simulink model "AutonomousModel_V3"  (R2020b)
settings: Solver=ode23t  StartTime=0.0  StopTime=180.1  FixedStep=0.05  RelTol=1e-3  EnableMultiTasking=on
model workspace (MAT data in the model file):
  mapForSim : object (value not decoded)
  occGrid : robotics.BinaryOccupancyGrid (value not decoded)
undefined symbols (not defined in the file): cellLevel, cellPose, cellTypeArray, FloorSurface, isoPoses, platformPoses, PlowSurface, Ref, RobotSurface, WallSurface, X, Y, Z
libraries: sm_lib x286, nesl_utility x157, simulink x72, pid_lib x3
(part 14 of 14)

== matlab function AutonomousModel_V3/BEST Robotics 2020 Game (Double-Click)/Cells/Object9/MATLAB Function ==
  settings: updateMethod=DISCRETE
  data: latch input; scoreLevel input; inuse input; target input; time input; objPoseX output; robotPoseX input; robotPoseY input; objPoseY output; latched output; initPose parameter; objId parameter; cellType output; endType output; cellTypeArray parameter; gameTime parameter; platformPoses parameter; cellLevel parameter
function [objPoseX, objPoseY, latched, cellType,endType] = latchObject(latch,scoreLevel, inuse, target, time, robotPoseX, robotPoseY, initPose, objId, cellTypeArray, gameTime, platformPoses, cellLevel)
persistent stateX stateY level pickup
if isempty(stateX)
    stateX=initPose(1);
    stateY=initPose(2);
    level=cellLevel;
    pickup=0;
end

if ~latch
     pickup=0;
    if level && ((stateX > platformPoses(1,1)-0.21 && stateX < platformPoses(1,1)+0.21...
            && stateY > platformPoses(1,2)-0.21 && stateY < platformPoses(1,2) +0.21) || ...
            (stateX > platformPoses(2,1)-0.21 && stateX < platformPoses(2,1)+0.21...
            && stateY > platformPoses(2,2)-0.21 && stateY < platformPoses(2,2) +0.21))
        latched=0.4;
    else
        level=0;
        latched=0;
    end
elseif pickup
    stateX=robotPoseX;
    stateY=robotPoseY;
    level=scoreLevel;
    latched=0.15 +level*0.4;
elseif ~inuse && latch && target == objId && ...
        sqrt((stateX-robotPoseX)^2+(stateY-robotPoseY)^2) < 0.08 && scoreLevel==level
    
        pickup=1;
        latched=0.15;
else
   if level && ((stateX > platformPoses(1,1)-0.21 && stateX < platformPoses(1,1)+0.21...
            && stateY > platformPoses(1,2)-0.21 && stateY < platformPoses(1,2) +0.21) || ...
            (stateX > platformPoses(2,1)-0.21 && stateX < platformPoses(2,1)+0.21...
            && stateY > platformPoses(2,2)-0.21 && stateY < platformPoses(2,2) +0.21))
        latched=0.4;
    else
        level=0;
        latched=0;
    end
end
if sqrt((stateX-robotPoseX)^2+(stateY-robotPoseY)^2) < 0.1 && scoreLevel==level
    cellType=cellTypeArray(objId);
else
    cellType=nan;
end

if time > gameTime
    endType=cellTypeArray(objId)+1;
else
    endType=0;
end

objPoseX=stateX;
objPoseY=stateY;

== stateflow chart AutonomousModel_V3/Stateflow ==
  state DROP_1
    entry: dropVac = [1 0 0]
  state DROP_2
    entry: dropVac = [0 1 1]
  state DROP_3
    entry: dropVac = [0 0 1]
  (default) -> DROP_1
  DROP_1 -> DROP_2 : after(1, sec)
  DROP_2 -> DROP_3 : after(1, sec)
  data: dropVac output

== stateflow chart AutonomousModel_V3/Simulink Function2/Stateflow2 ==
  state SETTLE
  state RESET_MOTORS
    entry:
    leftMotor = 0
    rightMotor = 0
  (default) -> SETTLE
  RESET_MOTORS -> SETTLE
  SETTLE -> RESET_MOTORS : [angleHasSettled]
  data: angleHasSettled input; leftMotor data_store_memory; rightMotor data_store_memory

== matlab function AutonomousModel_V3/BEST Robotics 2020 Game (Double-Click)/Cells/Object10/MATLAB Function ==
  settings: updateMethod=DISCRETE
  data: latch input; scoreLevel input; inuse input; target input; time input; objPoseX output; robotPoseX input; robotPoseY input; objPoseY output; latched output; initPose parameter; objId parameter; cellType output; endType output; cellTypeArray parameter; gameTime parameter; platformPoses parameter; cellLevel parameter
function [objPoseX, objPoseY, latched, cellType,endType] = latchObject(latch,scoreLevel, inuse, target, time, robotPoseX, robotPoseY, initPose, objId, cellTypeArray, gameTime, platformPoses, cellLevel)
persistent stateX stateY level pickup
if isempty(stateX)
    stateX=initPose(1);
    stateY=initPose(2);
    level=cellLevel;
    pickup=0;
end

if ~latch
     pickup=0;
    if level && ((stateX > platformPoses(1,1)-0.21 && stateX < platformPoses(1,1)+0.21...
            && stateY > platformPoses(1,2)-0.21 && stateY < platformPoses(1,2) +0.21) || ...
            (stateX > platformPoses(2,1)-0.21 && stateX < platformPoses(2,1)+0.21...
            && stateY > platformPoses(2,2)-0.21 && stateY < platformPoses(2,2) +0.21))
        latched=0.4;
    else
        level=0;
        latched=0;
    end
elseif pickup
    stateX=robotPoseX;
    stateY=robotPoseY;
    level=scoreLevel;
    latched=0.15 +level*0.4;
elseif ~inuse && latch && target == objId && ...
        sqrt((stateX-robotPoseX)^2+(stateY-robotPoseY)^2) < 0.08 && scoreLevel==level
    
        pickup=1;
        latched=0.15;
else
   if level && ((stateX > platformPoses(1,1)-0.21 && stateX < platformPoses(1,1)+0.21...
            && stateY > platformPoses(1,2)-0.21 && stateY < platformPoses(1,2) +0.21) || ...
            (stateX > platformPoses(2,1)-0.21 && stateX < platformPoses(2,1)+0.21...
            && stateY > platformPoses(2,2)-0.21 && stateY < platformPoses(2,2) +0.21))
        latched=0.4;
    else
        level=0;
        latched=0;
    end
end
if sqrt((stateX-robotPoseX)^2+(stateY-robotPoseY)^2) < 0.1 && scoreLevel==level
    cellType=cellTypeArray(objId);
else
    cellType=nan;
end

if time > gameTime
    endType=cellTypeArray(objId)+1;
else
    endType=0;
end

objPoseX=stateX;
objPoseY=stateY;

== matlab function AutonomousModel_V3/BEST Robotics 2020 Game (Double-Click)/Cells/Object11/MATLAB Function ==
  settings: updateMethod=DISCRETE
  data: latch input; scoreLevel input; inuse input; target input; time input; objPoseX output; robotPoseX input; robotPoseY input; objPoseY output; latched output; initPose parameter; objId parameter; cellType output; endType output; cellTypeArray parameter; gameTime parameter; platformPoses parameter; cellLevel parameter
function [objPoseX, objPoseY, latched, cellType,endType] = latchObject(latch,scoreLevel, inuse, target, time, robotPoseX, robotPoseY, initPose, objId, cellTypeArray, gameTime, platformPoses, cellLevel)
persistent stateX stateY level pickup
if isempty(stateX)
    stateX=initPose(1);
    stateY=initPose(2);
    level=cellLevel;
    pickup=0;
end

if ~latch
     pickup=0;
    if level && ((stateX > platformPoses(1,1)-0.21 && stateX < platformPoses(1,1)+0.21...
            && stateY > platformPoses(1,2)-0.21 && stateY < platformPoses(1,2) +0.21) || ...
            (stateX > platformPoses(2,1)-0.21 && stateX < platformPoses(2,1)+0.21...
            && stateY > platformPoses(2,2)-0.21 && stateY < platformPoses(2,2) +0.21))
        latched=0.4;
    else
        level=0;
        latched=0;
    end
elseif pickup
    stateX=robotPoseX;
    stateY=robotPoseY;
    level=scoreLevel;
    latched=0.15 +level*0.4;
elseif ~inuse && latch && target == objId && ...
        sqrt((stateX-robotPoseX)^2+(stateY-robotPoseY)^2) < 0.08 && scoreLevel==level
    
        pickup=1;
        latched=0.15;
else
   if level && ((stateX > platformPoses(1,1)-0.21 && stateX < platformPoses(1,1)+0.21...
            && stateY > platformPoses(1,2)-0.21 && stateY < platformPoses(1,2) +0.21) || ...
            (stateX > platformPoses(2,1)-0.21 && stateX < platformPoses(2,1)+0.21...
            && stateY > platformPoses(2,2)-0.21 && stateY < platformPoses(2,2) +0.21))
        latched=0.4;
    else
        level=0;
        latched=0;
    end
end
if sqrt((stateX-robotPoseX)^2+(stateY-robotPoseY)^2) < 0.1 && scoreLevel==level
    cellType=cellTypeArray(objId);
else
    cellType=nan;
end

if time > gameTime
    endType=cellTypeArray(objId)+1;
else
    endType=0;
end

objPoseX=stateX;
objPoseY=stateY;

== matlab function AutonomousModel_V3/BEST Robotics 2020 Game (Double-Click)/Cells/Object12/MATLAB Function ==
  settings: updateMethod=DISCRETE
  data: latch input; scoreLevel input; inuse input; target input; time input; objPoseX output; robotPoseX input; robotPoseY input; objPoseY output; latched output; initPose parameter; objId parameter; cellType output; endType output; cellTypeArray parameter; gameTime parameter; platformPoses parameter; cellLevel parameter
function [objPoseX, objPoseY, latched, cellType,endType] = latchObject(latch,scoreLevel, inuse, target, time, robotPoseX, robotPoseY, initPose, objId, cellTypeArray, gameTime, platformPoses, cellLevel)
persistent stateX stateY level pickup
if isempty(stateX)
    stateX=initPose(1);
    stateY=initPose(2);
    level=cellLevel;
    pickup=0;
end

if ~latch
     pickup=0;
    if level && ((stateX > platformPoses(1,1)-0.21 && stateX < platformPoses(1,1)+0.21...
            && stateY > platformPoses(1,2)-0.21 && stateY < platformPoses(1,2) +0.21) || ...
            (stateX > platformPoses(2,1)-0.21 && stateX < platformPoses(2,1)+0.21...
            && stateY > platformPoses(2,2)-0.21 && stateY < platformPoses(2,2) +0.21))
        latched=0.4;
    else
        level=0;
        latched=0;
    end
elseif pickup
    stateX=robotPoseX;
    stateY=robotPoseY;
    level=scoreLevel;
    latched=0.15 +level*0.4;
elseif ~inuse && latch && target == objId && ...
        sqrt((stateX-robotPoseX)^2+(stateY-robotPoseY)^2) < 0.08 && scoreLevel==level
    
        pickup=1;
        latched=0.15;
else
   if level && ((stateX > platformPoses(1,1)-0.21 && stateX < platformPoses(1,1)+0.21...
            && stateY > platformPoses(1,2)-0.21 && stateY < platformPoses(1,2) +0.21) || ...
            (stateX > platformPoses(2,1)-0.21 && stateX < platformPoses(2,1)+0.21...
            && stateY > platformPoses(2,2)-0.21 && stateY < platformPoses(2,2) +0.21))
        latched=0.4;
    else
        level=0;
        latched=0;
    end
end
if sqrt((stateX-robotPoseX)^2+(stateY-robotPoseY)^2) < 0.1 && scoreLevel==level
    cellType=cellTypeArray(objId);
else
    cellType=nan;
end

if time > gameTime
    endType=cellTypeArray(objId)+1;
else
    endType=0;
end

objPoseX=stateX;
objPoseY=stateY;

== matlab function AutonomousModel_V3/BEST Robotics 2020 Game (Double-Click)/Cells/Object13/MATLAB Function ==
  settings: updateMethod=DISCRETE
  data: latch input; scoreLevel input; inuse input; target input; time input; objPoseX output; robotPoseX input; robotPoseY input; objPoseY output; latched output; initPose parameter; objId parameter; cellType output; endType output; cellTypeArray parameter; gameTime parameter; platformPoses parameter; cellLevel parameter
function [objPoseX, objPoseY, latched, cellType,endType] = latchObject(latch,scoreLevel, inuse, target, time, robotPoseX, robotPoseY, initPose, objId, cellTypeArray, gameTime, platformPoses, cellLevel)
persistent stateX stateY level pickup
if isempty(stateX)
    stateX=initPose(1);
    stateY=initPose(2);
    level=cellLevel;
    pickup=0;
end

if ~latch
     pickup=0;
    if level && ((stateX > platformPoses(1,1)-0.21 && stateX < platformPoses(1,1)+0.21...
            && stateY > platformPoses(1,2)-0.21 && stateY < platformPoses(1,2) +0.21) || ...
            (stateX > platformPoses(2,1)-0.21 && stateX < platformPoses(2,1)+0.21...
            && stateY > platformPoses(2,2)-0.21 && stateY < platformPoses(2,2) +0.21))
        latched=0.4;
    else
        level=0;
        latched=0;
    end
elseif pickup
    stateX=robotPoseX;
    stateY=robotPoseY;
    level=scoreLevel;
    latched=0.15 +level*0.4;
elseif ~inuse && latch && target == objId && ...
        sqrt((stateX-robotPoseX)^2+(stateY-robotPoseY)^2) < 0.08 && scoreLevel==level
    
        pickup=1;
        latched=0.15;
else
   if level && ((stateX > platformPoses(1,1)-0.21 && stateX < platformPoses(1,1)+0.21...
            && stateY > platformPoses(1,2)-0.21 && stateY < platformPoses(1,2) +0.21) || ...
            (stateX > platformPoses(2,1)-0.21 && stateX < platformPoses(2,1)+0.21...
            && stateY > platformPoses(2,2)-0.21 && stateY < platformPoses(2,2) +0.21))
        latched=0.4;
    else
        level=0;
        latched=0;
    end
end
if sqrt((stateX-robotPoseX)^2+(stateY-robotPoseY)^2) < 0.1 && scoreLevel==level
    cellType=cellTypeArray(objId);
else
    cellType=nan;
end

if time > gameTime
    endType=cellTypeArray(objId)+1;
else
    endType=0;
end

objPoseX=stateX;
objPoseY=stateY;

== matlab function AutonomousModel_V3/BEST Robotics 2020 Game (Double-Click)/Cells/Object14/MATLAB Function ==
  settings: updateMethod=DISCRETE
  data: latch input; scoreLevel input; inuse input; target input; time input; objPoseX output; robotPoseX input; robotPoseY input; objPoseY output; latched output; initPose parameter; objId parameter; cellType output; endType output; cellTypeArray parameter; gameTime parameter; platformPoses parameter; cellLevel parameter
function [objPoseX, objPoseY, latched, cellType,endType] = latchObject(latch,scoreLevel, inuse, target, time, robotPoseX, robotPoseY, initPose, objId, cellTypeArray, gameTime, platformPoses, cellLevel)
persistent stateX stateY level pickup
if isempty(stateX)
    stateX=initPose(1);
    stateY=initPose(2);
    level=cellLevel;
    pickup=0;
end

if ~latch
     pickup=0;
    if level && ((stateX > platformPoses(1,1)-0.21 && stateX < platformPoses(1,1)+0.21...
            && stateY > platformPoses(1,2)-0.21 && stateY < platformPoses(1,2) +0.21) || ...
            (stateX > platformPoses(2,1)-0.21 && stateX < platformPoses(2,1)+0.21...
            && stateY > platformPoses(2,2)-0.21 && stateY < platformPoses(2,2) +0.21))
        latched=0.4;
    else
        level=0;
        latched=0;
    end
elseif pickup
    stateX=robotPoseX;
    stateY=robotPoseY;
    level=scoreLevel;
    latched=0.15 +level*0.4;
elseif ~inuse && latch && target == objId && ...
        sqrt((stateX-robotPoseX)^2+(stateY-robotPoseY)^2) < 0.08 && scoreLevel==level
    
        pickup=1;
        latched=0.15;
else
   if level && ((stateX > platformPoses(1,1)-0.21 && stateX < platformPoses(1,1)+0.21...
            && stateY > platformPoses(1,2)-0.21 && stateY < platformPoses(1,2) +0.21) || ...
            (stateX > platformPoses(2,1)-0.21 && stateX < platformPoses(2,1)+0.21...
            && stateY > platformPoses(2,2)-0.21 && stateY < platformPoses(2,2) +0.21))
        latched=0.4;
    else
        level=0;
        latched=0;
    end
end
if sqrt((stateX-robotPoseX)^2+(stateY-robotPoseY)^2) < 0.1 && scoreLevel==level
    cellType=cellTypeArray(objId);
else
    cellType=nan;
end

if time > gameTime
    endType=cellTypeArray(objId)+1;
else
    endType=0;
end

objPoseX=stateX;
objPoseY=stateY;

== matlab function AutonomousModel_V3/BEST Robotics 2020 Game (Double-Click)/Cells/Object15/MATLAB Function ==
  settings: updateMethod=DISCRETE
  data: latch input; scoreLevel input; inuse input; target input; time input; objPoseX output; robotPoseX input; robotPoseY input; objPoseY output; latched output; initPose parameter; objId parameter; cellType output; endType output; cellTypeArray parameter; gameTime parameter; platformPoses parameter; cellLevel parameter
function [objPoseX, objPoseY, latched, cellType,endType] = latchObject(latch,scoreLevel, inuse, target, time, robotPoseX, robotPoseY, initPose, objId, cellTypeArray, gameTime, platformPoses, cellLevel)
persistent stateX stateY level pickup
if isempty(stateX)
    stateX=initPose(1);
    stateY=initPose(2);
    level=cellLevel;
    pickup=0;
end

if ~latch
     pickup=0;
    if level && ((stateX > platformPoses(1,1)-0.21 && stateX < platformPoses(1,1)+0.21...
            && stateY > platformPoses(1,2)-0.21 && stateY < platformPoses(1,2) +0.21) || ...
            (stateX > platformPoses(2,1)-0.21 && stateX < platformPoses(2,1)+0.21...
            && stateY > platformPoses(2,2)-0.21 && stateY < platformPoses(2,2) +0.21))
        latched=0.4;
    else
        level=0;
        latched=0;
    end
elseif pickup
    stateX=robotPoseX;
    stateY=robotPoseY;
    level=scoreLevel;
    latched=0.15 +level*0.4;
elseif ~inuse && latch && target == objId && ...
        sqrt((stateX-robotPoseX)^2+(stateY-robotPoseY)^2) < 0.08 && scoreLevel==level
    
        pickup=1;
        latched=0.15;
else
   if level && ((stateX > platformPoses(1,1)-0.21 && stateX < platformPoses(1,1)+0.21...
            && stateY > platformPoses(1,2)-0.21 && stateY < platformPoses(1,2) +0.21) || ...
            (stateX > platformPoses(2,1)-0.21 && stateX < platformPoses(2,1)+0.21...
            && stateY > platformPoses(2,2)-0.21 && stateY < platformPoses(2,2) +0.21))
        latched=0.4;
    else
        level=0;
        latched=0;
    end
end
if sqrt((stateX-robotPoseX)^2+(stateY-robotPoseY)^2) < 0.1 && scoreLevel==level
    cellType=cellTypeArray(objId);
else
    cellType=nan;
end

if time > gameTime
    endType=cellTypeArray(objId)+1;
else
    endType=0;
end

objPoseX=stateX;
objPoseY=stateY;

== matlab function AutonomousModel_V3/BEST Robotics 2020 Game (Double-Click)/Cells/Object16/MATLAB Function ==
  settings: updateMethod=DISCRETE
  data: latch input; scoreLevel input; inuse input; target input; time input; objPoseX output; robotPoseX input; robotPoseY input; objPoseY output; latched output; initPose parameter; objId parameter; cellType output; endType output; cellTypeArray parameter; gameTime parameter; platformPoses parameter; cellLevel parameter
function [objPoseX, objPoseY, latched, cellType,endType] = latchObject(latch,scoreLevel, inuse, target, time, robotPoseX, robotPoseY, initPose, objId, cellTypeArray, gameTime, platformPoses, cellLevel)
persistent stateX stateY level pickup
if isempty(stateX)
    stateX=initPose(1);
    stateY=initPose(2);
    level=cellLevel;
    pickup=0;
end

if ~latch
     pickup=0;
    if level && ((stateX > platformPoses(1,1)-0.21 && stateX < platformPoses(1,1)+0.21...
            && stateY > platformPoses(1,2)-0.21 && stateY < platformPoses(1,2) +0.21) || ...
            (stateX > platformPoses(2,1)-0.21 && stateX < platformPoses(2,1)+0.21...
            && stateY > platformPoses(2,2)-0.21 && stateY < platformPoses(2,2) +0.21))
        latched=0.4;
    else
        level=0;
        latched=0;
    end
elseif pickup
    stateX=robotPoseX;
    stateY=robotPoseY;
    level=scoreLevel;
    latched=0.15 +level*0.4;
elseif ~inuse && latch && target == objId && ...
        sqrt((stateX-robotPoseX)^2+(stateY-robotPoseY)^2) < 0.08 && scoreLevel==level
    
        pickup=1;
        latched=0.15;
else
   if level && ((stateX > platformPoses(1,1)-0.21 && stateX < platformPoses(1,1)+0.21...
            && stateY > platformPoses(1,2)-0.21 && stateY < platformPoses(1,2) +0.21) || ...
            (stateX > platformPoses(2,1)-0.21 && stateX < platformPoses(2,1)+0.21...
            && stateY > platformPoses(2,2)-0.21 && stateY < platformPoses(2,2) +0.21))
        latched=0.4;
    else
        level=0;
        latched=0;
    end
end
if sqrt((stateX-robotPoseX)^2+(stateY-robotPoseY)^2) < 0.1 && scoreLevel==level
    cellType=cellTypeArray(objId);
else
    cellType=nan;
end

if time > gameTime
    endType=cellTypeArray(objId)+1;
else
    endType=0;
end

objPoseX=stateX;
objPoseY=stateY;

== matlab function AutonomousModel_V3/BEST Robotics 2020 Game (Double-Click)/Cells/Object17/MATLAB Function ==
  settings: updateMethod=DISCRETE
  data: latch input; scoreLevel input; inuse input; target input; time input; objPoseX output; robotPoseX input; robotPoseY input; objPoseY output; latched output; initPose parameter; objId parameter; cellType output; endType output; cellTypeArray parameter; gameTime parameter; platformPoses parameter; cellLevel parameter
function [objPoseX, objPoseY, latched, cellType,endType] = latchObject(latch,scoreLevel, inuse, target, time, robotPoseX, robotPoseY, initPose, objId, cellTypeArray, gameTime, platformPoses, cellLevel)
persistent stateX stateY level pickup
if isempty(stateX)
    stateX=initPose(1);
    stateY=initPose(2);
    level=cellLevel;
    pickup=0;
end

if ~latch
     pickup=0;
    if level && ((stateX > platformPoses(1,1)-0.21 && stateX < platformPoses(1,1)+0.21...
            && stateY > platformPoses(1,2)-0.21 && stateY < platformPoses(1,2) +0.21) || ...
            (stateX > platformPoses(2,1)-0.21 && stateX < platformPoses(2,1)+0.21...
            && stateY > platformPoses(2,2)-0.21 && stateY < platformPoses(2,2) +0.21))
        latched=0.4;
    else
        level=0;
        latched=0;
    end
elseif pickup
    stateX=robotPoseX;
    stateY=robotPoseY;
    level=scoreLevel;
    latched=0.15 +level*0.4;
elseif ~inuse && latch && target == objId && ...
        sqrt((stateX-robotPoseX)^2+(stateY-robotPoseY)^2) < 0.08 && scoreLevel==level
    
        pickup=1;
        latched=0.15;
else
   if level && ((stateX > platformPoses(1,1)-0.21 && stateX < platformPoses(1,1)+0.21...
            && stateY > platformPoses(1,2)-0.21 && stateY < platformPoses(1,2) +0.21) || ...
            (stateX > platformPoses(2,1)-0.21 && stateX < platformPoses(2,1)+0.21...
            && stateY > platformPoses(2,2)-0.21 && stateY < platformPoses(2,2) +0.21))
        latched=0.4;
    else
        level=0;
        latched=0;
    end
end
if sqrt((stateX-robotPoseX)^2+(stateY-robotPoseY)^2) < 0.1 && scoreLevel==level
    cellType=cellTypeArray(objId);
else
    cellType=nan;
end

if time > gameTime
    endType=cellTypeArray(objId)+1;
else
    endType=0;
end

objPoseX=stateX;
objPoseY=stateY;

== matlab function AutonomousModel_V3/BEST Robotics 2020 Game (Double-Click)/Cells/Object18/MATLAB Function ==
  settings: updateMethod=DISCRETE
  data: latch input; scoreLevel input; inuse input; target input; time input; objPoseX output; robotPoseX input; robotPoseY input; objPoseY output; latched output; initPose parameter; objId parameter; cellType output; endType output; cellTypeArray parameter; gameTime parameter; platformPoses parameter; cellLevel parameter
function [objPoseX, objPoseY, latched, cellType,endType] = latchObject(latch,scoreLevel, inuse, target, time, robotPoseX, robotPoseY, initPose, objId, cellTypeArray, gameTime, platformPoses, cellLevel)
persistent stateX stateY level pickup
if isempty(stateX)
    stateX=initPose(1);
    stateY=initPose(2);
    level=cellLevel;
    pickup=0;
end

if ~latch
     pickup=0;
    if level && ((stateX > platformPoses(1,1)-0.21 && stateX < platformPoses(1,1)+0.21...
            && stateY > platformPoses(1,2)-0.21 && stateY < platformPoses(1,2) +0.21) || ...
            (stateX > platformPoses(2,1)-0.21 && stateX < platformPoses(2,1)+0.21...
            && stateY > platformPoses(2,2)-0.21 && stateY < platformPoses(2,2) +0.21))
        latched=0.4;
    else
        level=0;
        latched=0;
    end
elseif pickup
    stateX=robotPoseX;
    stateY=robotPoseY;
    level=scoreLevel;
    latched=0.15 +level*0.4;
elseif ~inuse && latch && target == objId && ...
        sqrt((stateX-robotPoseX)^2+(stateY-robotPoseY)^2) < 0.08 && scoreLevel==level
    
        pickup=1;
        latched=0.15;
else
   if level && ((stateX > platformPoses(1,1)-0.21 && stateX < platformPoses(1,1)+0.21...
            && stateY > platformPoses(1,2)-0.21 && stateY < platformPoses(1,2) +0.21) || ...
            (stateX > platformPoses(2,1)-0.21 && stateX < platformPoses(2,1)+0.21...
            && stateY > platformPoses(2,2)-0.21 && stateY < platformPoses(2,2) +0.21))
        latched=0.4;
    else
        level=0;
        latched=0;
    end
end
if sqrt((stateX-robotPoseX)^2+(stateY-robotPoseY)^2) < 0.1 && scoreLevel==level
    cellType=cellTypeArray(objId);
else
    cellType=nan;
end

if time > gameTime
    endType=cellTypeArray(objId)+1;
else
    endType=0;
end

objPoseX=stateX;
objPoseY=stateY;

== matlab function AutonomousModel_V3/BEST Robotics 2020 Game (Double-Click)/Cells/Object19/MATLAB Function ==
  settings: updateMethod=DISCRETE
  data: latch input; scoreLevel input; inuse input; target input; time input; objPoseX output; robotPoseX input; robotPoseY input; objPoseY output; latched output; initPose parameter; objId parameter; cellType output; endType output; cellTypeArray parameter; gameTime parameter; platformPoses parameter; cellLevel parameter
function [objPoseX, objPoseY, latched, cellType,endType] = latchObject(latch,scoreLevel, inuse, target, time, robotPoseX, robotPoseY, initPose, objId, cellTypeArray, gameTime, platformPoses, cellLevel)
persistent stateX stateY level pickup
if isempty(stateX)
    stateX=initPose(1);
    stateY=initPose(2);
    level=cellLevel;
    pickup=0;
end

if ~latch
     pickup=0;
    if level && ((stateX > platformPoses(1,1)-0.21 && stateX < platformPoses(1,1)+0.21...
            && stateY > platformPoses(1,2)-0.21 && stateY < platformPoses(1,2) +0.21) || ...
            (stateX > platformPoses(2,1)-0.21 && stateX < platformPoses(2,1)+0.21...
            && stateY > platformPoses(2,2)-0.21 && stateY < platformPoses(2,2) +0.21))
        latched=0.4;
    else
        level=0;
        latched=0;
    end
elseif pickup
    stateX=robotPoseX;
    stateY=robotPoseY;
    level=scoreLevel;
    latched=0.15 +level*0.4;
elseif ~inuse && latch && target == objId && ...
        sqrt((stateX-robotPoseX)^2+(stateY-robotPoseY)^2) < 0.08 && scoreLevel==level
    
        pickup=1;
        latched=0.15;
else
   if level && ((stateX > platformPoses(1,1)-0.21 && stateX < platformPoses(1,1)+0.21...
            && stateY > platformPoses(1,2)-0.21 && stateY < platformPoses(1,2) +0.21) || ...
            (stateX > platformPoses(2,1)-0.21 && stateX < platformPoses(2,1)+0.21...
            && stateY > platformPoses(2,2)-0.21 && stateY < platformPoses(2,2) +0.21))
        latched=0.4;
    else
        level=0;
        latched=0;
    end
end
if sqrt((stateX-robotPoseX)^2+(stateY-robotPoseY)^2) < 0.1 && scoreLevel==level
    cellType=cellTypeArray(objId);
else
    cellType=nan;
end

if time > gameTime
    endType=cellTypeArray(objId)+1;
else
    endType=0;
end

objPoseX=stateX;
objPoseY=stateY;

== matlab function AutonomousModel_V3/BEST Robotics 2020 Game (Double-Click)/Cells/Object20/MATLAB Function ==
  settings: updateMethod=DISCRETE
  data: latch input; scoreLevel input; inuse input; target input; time input; objPoseX output; robotPoseX input; robotPoseY input; objPoseY output; latched output; initPose parameter; objId parameter; cellType output; endType output; cellTypeArray parameter; gameTime parameter; platformPoses parameter; cellLevel parameter
function [objPoseX, objPoseY, latched, cellType,endType] = latchObject(latch,scoreLevel, inuse, target, time, robotPoseX, robotPoseY, initPose, objId, cellTypeArray, gameTime, platformPoses, cellLevel)
persistent stateX stateY level pickup
if isempty(stateX)
    stateX=initPose(1);
    stateY=initPose(2);
    level=cellLevel;
    pickup=0;
end

if ~latch
     pickup=0;
    if level && ((stateX > platformPoses(1,1)-0.21 && stateX < platformPoses(1,1)+0.21...
            && stateY > platformPoses(1,2)-0.21 && stateY < platformPoses(1,2) +0.21) || ...
            (stateX > platformPoses(2,1)-0.21 && stateX < platformPoses(2,1)+0.21...
            && stateY > platformPoses(2,2)-0.21 && stateY < platformPoses(2,2) +0.21))
        latched=0.4;
    else
        level=0;
        latched=0;
    end
elseif pickup
    stateX=robotPoseX;
    stateY=robotPoseY;
    level=scoreLevel;
    latched=0.15 +level*0.4;
elseif ~inuse && latch && target == objId && ...
        sqrt((stateX-robotPoseX)^2+(stateY-robotPoseY)^2) < 0.08 && scoreLevel==level
    
        pickup=1;
        latched=0.15;
else
   if level && ((stateX > platformPoses(1,1)-0.21 && stateX < platformPoses(1,1)+0.21...
            && stateY > platformPoses(1,2)-0.21 && stateY < platformPoses(1,2) +0.21) || ...
            (stateX > platformPoses(2,1)-0.21 && stateX < platformPoses(2,1)+0.21...
            && stateY > platformPoses(2,2)-0.21 && stateY < platformPoses(2,2) +0.21))
        latched=0.4;
    else
        level=0;
        latched=0;
    end
end
if sqrt((stateX-robotPoseX)^2+(stateY-robotPoseY)^2) < 0.1 && scoreLevel==level
    cellType=cellTypeArray(objId);
else
    cellType=nan;
end

if time > gameTime
    endType=cellTypeArray(objId)+1;
else
    endType=0;
end

objPoseX=stateX;
objPoseY=stateY;

== matlab function AutonomousModel_V3/BEST Robotics 2020 Game (Double-Click)/Cells/Object21/MATLAB Function ==
  settings: updateMethod=DISCRETE
  data: latch input; scoreLevel input; inuse input; target input; time input; objPoseX output; robotPoseX input; robotPoseY input; objPoseY output; latched output; initPose parameter; objId parameter; cellType output; endType output; cellTypeArray parameter; gameTime parameter; platformPoses parameter; cellLevel parameter
function [objPoseX, objPoseY, latched, cellType,endType] = latchObject(latch,scoreLevel, inuse, target, time, robotPoseX, robotPoseY, initPose, objId, cellTypeArray, gameTime, platformPoses, cellLevel)
persistent stateX stateY level pickup
if isempty(stateX)
    stateX=initPose(1);
    stateY=initPose(2);
    level=cellLevel;
    pickup=0;
end

if ~latch
     pickup=0;
    if level && ((stateX > platformPoses(1,1)-0.21 && stateX < platformPoses(1,1)+0.21...
            && stateY > platformPoses(1,2)-0.21 && stateY < platformPoses(1,2) +0.21) || ...
            (stateX > platformPoses(2,1)-0.21 && stateX < platformPoses(2,1)+0.21...
            && stateY > platformPoses(2,2)-0.21 && stateY < platformPoses(2,2) +0.21))
        latched=0.4;
    else
        level=0;
        latched=0;
    end
elseif pickup
    stateX=robotPoseX;
    stateY=robotPoseY;
    level=scoreLevel;
    latched=0.15 +level*0.4;
elseif ~inuse && latch && target == objId && ...
        sqrt((stateX-robotPoseX)^2+(stateY-robotPoseY)^2) < 0.08 && scoreLevel==level
    
        pickup=1;
        latched=0.15;
else
   if level && ((stateX > platformPoses(1,1)-0.21 && stateX < platformPoses(1,1)+0.21...
            && stateY > platformPoses(1,2)-0.21 && stateY < platformPoses(1,2) +0.21) || ...
            (stateX > platformPoses(2,1)-0.21 && stateX < platformPoses(2,1)+0.21...
            && stateY > platformPoses(2,2)-0.21 && stateY < platformPoses(2,2) +0.21))
        latched=0.4;
    else
        level=0;
        latched=0;
    end
end
if sqrt((stateX-robotPoseX)^2+(stateY-robotPoseY)^2) < 0.1 && scoreLevel==level
    cellType=cellTypeArray(objId);
else
    cellType=nan;
end

if time > gameTime
    endType=cellTypeArray(objId)+1;
else
    endType=0;
end

objPoseX=stateX;
objPoseY=stateY;

== matlab function AutonomousModel_V3/BEST Robotics 2020 Game (Double-Click)/Cells/MATLAB Function2 ==
  data: robotPose input; cellPoses input; cellTarget output
function cellTarget = findTarget(robotPose, cellPoses)


eucDist=sqrt((cellPoses(:,1)-robotPose(1)).^2+(cellPoses(:,2)-robotPose(2)).^2);
[~,cellIdx]=min(eucDist);
cellTarget = cellIdx;

== matlab function AutonomousModel_V3/BEST Robotics 2020 Game (Double-Click)/Vaccines/Vaccine/MATLAB Function ==
  settings: updateMethod=DISCRETE
  data: drop input; level input; objPoseX output; robotPoseX input; robotPoseY input; objPoseY output; vaccine output
function [objPoseX, objPoseY, vaccine] = latchObject(drop, level, robotPoseX, robotPoseY)
persistent stateX stateY stateZ prevDrop dropped
if isempty(stateX)
    stateX=robotPoseX+0.14;
    stateY=robotPoseY;
    stateZ=0.15;
    prevDrop=0;
    dropped=0;
end

if drop && prevDrop && ~dropped
    stateX=robotPoseX;
    stateY=robotPoseY;
    stateZ=level*0.4;
    objPoseX=robotPoseX;
    objPoseY=robotPoseY;
    dropped=1;
elseif dropped
    objPoseX=stateX;
    objPoseY=stateY;

else
    objPoseX=robotPoseX+0.14;
    objPoseY=robotPoseY;
end
prevDrop=drop;
vaccine=stateZ;

== matlab function AutonomousModel_V3/BEST Robotics 2020 Game (Double-Click)/Vaccines/Vaccine2/MATLAB Function1 ==
  settings: updateMethod=DISCRETE
  data: drop input; level input; objPoseX output; robotPoseX input; robotPoseY input; objPoseY output; vaccine output
function [objPoseX, objPoseY, vaccine] = latchObject(drop, level, robotPoseX, robotPoseY)
persistent stateX stateY stateZ prevDrop dropped
if isempty(stateX)
    stateX=robotPoseX+0.14;
    stateY=robotPoseY;
    stateZ=0.15;
    prevDrop=0;
    dropped=0;
end

if drop && prevDrop && ~dropped
    stateX=robotPoseX;
    stateY=robotPoseY;
    stateZ=level*0.4;
    objPoseX=robotPoseX;
    objPoseY=robotPoseY;
    dropped=1;
elseif dropped
    objPoseX=stateX;
    objPoseY=stateY;

else
    objPoseX=robotPoseX-0.11;
    objPoseY=robotPoseY+0.11;
end
prevDrop=drop;
vaccine=stateZ;

== stateflow chart AutonomousModel_V3/Stateflow3 ==
  state MAIN_PROGRAM [commented out]
    state PAHSE_2 [commented out]
    state PHASE_1 [commented out]
      state deliveredVac = hasDroppedVacAt(xCoord, yCoord) [function] [commented out]
      state DROP_VAC_1 [commented out]
      state DROP_VAC_2 [commented out]
      state platformCleared = hasClearedPlatformAt(gridX, gridY) [function] [commented out]
      state CLEAR_PLATFORM_1 [commented out]
      note: Discrete grid-square system coordinates
      state DROP_VAC_3 [commented out]
      state CLEAR_PLATFORM_2 [commented out]
      (default) -> DROP_VAC_1 [commented out]
      DROP_VAC_1 -> DROP_VAC_2 [commented out] : [hasDroppedVacAt(1.066667, 0.761905)]
      DROP_VAC_2 -> CLEAR_PLATFORM_1 [commented out] : [hasDroppedVacAt(1.066667, 2.438095)]
      CLEAR_PLATFORM_1 -> DROP_VAC_3 [commented out] : [hasClearedPlatformAt(5, 5)]
      DROP_VAC_3 -> CLEAR_PLATFORM_2 [commented out] : [hasDroppedVacAt(2.514286, 1.676190)]
    (default) -> PHASE_1 [commented out]
    CLEAR_PLATFORM_2 -> PAHSE_2 [commented out] : [hasClearedPlatformAt(6, 0)]
  state TEST_PROGRAM
    state MOVE_TO_GRID
    state MOVE_TO_GRID1
    state MOVE_TO_GRID2
    state DONE
      entry:
      leftMotor = -127
      rightMotor = 127
    (default) -> MOVE_TO_GRID
    MOVE_TO_GRID1 -> MOVE_TO_GRID2 : [hasMovedToCoords(0, 0)]
    MOVE_TO_GRID -> MOVE_TO_GRID1 : [hasMovedToCoords(3.2, 1.6)]
    MOVE_TO_GRID2 -> DONE : [hasMovedToCoords(1.6, 1.6)]
  (default) -> MAIN_PROGRAM [commented out]
  data: xCoord function_input double size=1; yCoord function_input double size=1; deliveredVac function_output double size=1; gridX function_input double size=1; gridY function_input double size=1; platformCleared function_output double size=1; leftMotor data_store_memory; rightMotor data_store_memory

== matlab function AutonomousModel_V3/BEST Robotics 2020 Game (Double-Click)/Vaccines/Vaccine1/MATLAB Function1 ==
  settings: updateMethod=DISCRETE
  data: drop input; level input; objPoseX output; robotPoseX input; robotPoseY input; objPoseY output; vaccine output
function [objPoseX, objPoseY, vaccine] = latchObject(drop, level, robotPoseX, robotPoseY)
persistent stateX stateY stateZ prevDrop dropped
if isempty(stateX)
    stateX=robotPoseX+0.14;
    stateY=robotPoseY;
    stateZ=0.15;
    prevDrop=0;
    dropped=0;
end

if drop && prevDrop && ~dropped
    stateX=robotPoseX;
    stateY=robotPoseY;
    stateZ=level*0.4;
    objPoseX=robotPoseX;
    objPoseY=robotPoseY;
    dropped=1;
elseif dropped
    objPoseX=stateX;
    objPoseY=stateY;

else
    objPoseX=robotPoseX-0.11;
    objPoseY=robotPoseY-0.11;
end
prevDrop=drop;
vaccine=stateZ;

== matlab function AutonomousModel_V3/MATLAB Function1 ==
  data: fullRobotAngle input; fullRobotAngle output; leftTicks input; rightTicks input; prevLTicks input; prevRTicks input
function fullRobotAngle = getFullRobotAngle(fullRobotAngle, ...
    leftTicks, rightTicks, prevLTicks, prevRTicks)

% just choose one of the encoder tick differences, since
    % the motors always have the same speed
% the weird decimal is the change in degrees per encoder tick
angleChange = abs(leftTicks - prevLTicks) * 0.7804878049;

% if the robot is turning clockwise
if leftTicks > prevLTicks && rightTicks < prevRTicks
    fullRobotAngle = fullRobotAngle - angleChange;
% if the robot is turning counter-clockwise
elseif rightTicks > prevRTicks && leftTicks < prevLTicks
    fullRobotAngle = fullRobotAngle + angleChange;
end

% normalize the angle to be 0 to 359 degrees
if fullRobotAngle >= 360
    fullRobotAngle = mod(fullRobotAngle, 360);
elseif fullRobotAngle < 0
    fullRobotAngle = fullRobotAngle + 360;
end

== stateflow chart AutonomousModel_V3/Stateflow3/MAIN_PROGRAM.PHASE_1.hasDroppedVacAt/Stateflow ==
  state DROP_VACCINE
    entry:
    leftMotor = 0
    rightMotor = 0
    %dropVaccine()
    vaccineDropped = true
  state MOVE_TO_VAC_SQUARE
  (default) -> MOVE_TO_VAC_SQUARE
  MOVE_TO_VAC_SQUARE -> DROP_VACCINE : [hasMovedToCoords(xCoord, yCoord)]
  data: xCoord input; yCoord input; vaccineDropped output; leftMotor data_store_memory; rightMotor data_store_memory

== stateflow chart AutonomousModel_V3/Simulink Function2/Stateflow ==
  state ELAPSE_SETTLE_TIME
    during:
    settledTime = settledTime + 1
  state RESET_SETTLE_TIME
    entry:
    settledTime = 0
  (default) -> RESET_SETTLE_TIME
  RESET_SETTLE_TIME -> ELAPSE_SETTLE_TIME : [error <= TOLERANCE]
  ELAPSE_SETTLE_TIME -> RESET_SETTLE_TIME : [error > TOLERANCE]
  data: TOLERANCE input; error input; settledTime data_store_memory

== stateflow chart AutonomousModel_V3/Simulink Function3/Stateflow1 ==
  state CALCULATE_PATH
    entry:
    hasArrived = false
    changeX = xCoord - xPos
    changeY = yCoord - yPos
    targetAngle = normalizeAngle(...
    atand(changeY / changeX), changeX)
    targetDist = sqrt(changeX^2 + changeY^2) - 0.2699019608
    oldXCoord = xCoord
    oldYCoord = yCoord
  state TURN_TO_TARGET
  state DRIVE_TO_TARGET
  state HAS_ARRIVED
    entry: hasArrived = true
  (default) -> CALCULATE_PATH
  CALCULATE_PATH -> TURN_TO_TARGET
  TURN_TO_TARGET -> DRIVE_TO_TARGET : [hasTurnedToAngle(targetAngle)]
  DRIVE_TO_TARGET -> HAS_ARRIVED : [hasMovedDist(targetDist)]
  HAS_ARRIVED -> CALCULATE_PATH : [xCoord ~= oldXCoord || yCoord ~= oldYCoord]
  data: angle function_output; angle function_input; xChange function_input; xCoord input; yCoord input; targetDist local; targetAngle local; xPos data_store_memory; yPos data_store_memory; hasArrived output; oldYCoord local; oldXCoord local; changeY local; changeX local
  function angle = normalizeAngle(angle, xChange):
    | function angle = normalizeAngle(angle, xChange)
    | 
    | if xChange < 0
    |     angle = angle + 180;
    | end

== stateflow chart AutonomousModel_V3/Simulink Function1/Stateflow ==
  state SETTLE
  state RESET_DIST_AFTER_SETTLE
    entry:
    leftMotor = 0
    rightMotor = 0
    resetLeftEncoder = 1
    resetRightEncoder = 1
    straightDistTraveled = 0
    resetLeftEncoder = 0
    resetRightEncoder = 0
  (default) -> SETTLE
  RESET_DIST_AFTER_SETTLE -> SETTLE
  SETTLE -> RESET_DIST_AFTER_SETTLE : [distHasSettled]
  data: distHasSettled input; resetLeftEncoder data_store_memory; resetRightEncoder data_store_memory; straightDistTraveled data_store_memory; leftMotor data_store_memory; rightMotor data_store_memory

== matlab function AutonomousModel_V3/Simulink Function1/MATLAB Function ==
  data: u input double size=1; sign output double size=1
function sign = fcn(u)

if u > 0
    sign = 1;
elseif u < 0
    sign = -1;
else
    sign = 0;
end

== stateflow chart AutonomousModel_V3/Simulink Function1/Stateflow1 ==
  state ELAPSE_SETTLE_TIME
    during:
    settledTime = settledTime + 1
  state RESET_SETTLE_TIME
    entry:
    settledTime = 0
  (default) -> RESET_SETTLE_TIME
  RESET_SETTLE_TIME -> ELAPSE_SETTLE_TIME : [error <= TOLERANCE]
  ELAPSE_SETTLE_TIME -> RESET_SETTLE_TIME : [error > TOLERANCE]
  data: TOLERANCE input; error input; settledTime data_store_memory

== stateflow chart AutonomousModel_V3/Simulink Function4/Stateflow1 ==
  (default) -> (junction 11)
  (junction 11) -> (junction 12) [order 1] : [all((vaccineReleases == [0 0 0]) == 1)]
  (junction 11) -> (junction 13) [order 2]
  (junction 12) -> (junction 17) : {vaccineReleases = [1 0 0];}
  (junction 13) -> (junction 14) [order 1] : [all((vaccineReleases == [1 0 0]) == 1)]
  (junction 13) -> (junction 15) [order 2] : {vaccineReleases = [1 1 1];}
  (junction 14) -> (junction 16) : {vaccineReleases = [1 1 0];}
  (junction 16) -> (junction 15)
  (junction 17) -> (junction 16)
  data: vaccineReleases data_store_memory

== matlab function AutonomousModel_V3/MATLAB Function ==
  data: changeInDist input; fullRobotAngle input; deltaX output; deltaY output
function [deltaX, deltaY] = getCoordChanges(changeInDist, fullRobotAngle)
% assumes that the robot angle input is from 0 to 360 degrees

deltaX = changeInDist * cosd(fullRobotAngle);
deltaY = changeInDist * sind(fullRobotAngle);

== matlab function AutonomousModel_V3/MATLAB Function2 ==
  data: fullRobotAngle input; latchXPos output; robotXPos input; robotYPos input; latchYPos output
function [latchXPos, latchYPos] = getLatchPos(fullRobotAngle, robotXPos, robotYPos)
% the weird decimal number is the const final constant distance
% between the robot's (x, y) and its latcher's (x, y)
latchXPos = robotXPos + 0.3812987013*cosd(fullRobotAngle);
latchYPos = robotYPos + 0.3812987013*sind(fullRobotAngle);

== matlab function AutonomousModel_V3/MATLAB Function3 ==
  data: leftTicks input; distChange output; rightTicks input; prevLTicks input; prevRTicks input; moveDir input; prevLTicks output; prevRTicks output
function [distChange, prevLTicks, prevRTicks] = getDistChange(leftTicks, rightTicks, ...
    prevLTicks, prevRTicks, moveDir)

% weird decimal is 0.5 * TICKS_TO_DIST, where TICKS_TO_DIST = (2*pi*0.1) / 180
distChange = ((leftTicks - prevLTicks) + (rightTicks - prevRTicks)) ...
    * (moveDir * 0.00174532925);

prevLTicks = leftTicks;
prevRTicks = rightTicks;

== matlab function AutonomousModel_V3/Simulink Function2/MATLAB Function1 ==
  data: angleDiff input; optimalAngleDiff output
function optimalAngleDiff = filterErrorAngle(angleDiff)

if abs(angleDiff) > 180
    if angleDiff < 0
        optimalAngleDiff = angleDiff + 360;
    else
        optimalAngleDiff = angleDiff - 360;
    end
else
    optimalAngleDiff = angleDiff;
end

== matlab function AutonomousModel_V3/Simulink Function2/MATLAB Function2 ==
  data: targetAngle input; targetAngle output
function targetAngle = fixUserAngle(targetAngle)

% angle wrapper function to fix user input angle assumes
% an extreme input from -360 to 360

if targetAngle < 0 || targetAngle > 359
    targetAngle = mod(targetAngle, 360);
end

== matlab function AutonomousModel_V3/MATLAB Function4 ==
  data: cellType input; green output; orange output; red output
function [green, orange, red] = displayCellType(cellType)

green = 0;
orange = 0;
red = 0;

% Identify the detected cell type and lit up the corresponding lamp bit
if ~isnan(cellType)
    switch cellType
        case 0
            orange = 1;
        case 1
            green = 1;
        case 2
            red = 1;
    end   
end
